simulink model "kukaXYZctrl"  (R2016b)
settings: Solver=ode5  StartTime=0.0  StopTime=inf  FixedStep=0.001  RelTol=1e-3  EnableMultiTasking=on
undefined symbols (not defined in the file): Standard_Devices, UDP_Protocol
libraries: dcpctrl x2, kukaslxctrl x1, sldrtlib x1, simulink x1
settings Model: SimulationMode=external  Creator=julianleland  LastModifiedBy=julianleland
settings OptimizationCC: LifeSpan=inf
settings DebuggingCC: SFUnexpectedBacktrackingDiag=warning  SFNoUnconditionalDefaultTransitionDiag=warning  SFExecutionAtInitializationDiag=none
settings HardwareCC: ProdBitPerLong=64  ProdHWDeviceType=Intel->x86-64 (Mac OS X)  TargetBitPerLong=64  TargetBitPerPointer=64  TargetIntDivRoundTo=Zero  TargetEndianess=LittleEndian  TargetWordSize=64  TargetHWDeviceType=Intel->x86-64
settings RTWCC: SystemTargetFile=sldrt.tlc  TemplateMakefile=sldrt.tmf  Description=Simulink Desktop Real-Time  RTWCompilerOptimization=on
settings CodeAppCC: MaxIdLength=95
settings SimulinkDesktopRealTimeCC: TargetPreCompLibLocation=/Applications/MATLAB_R2016b.app/toolbox/sldrt/lib/maci64  TargetLangStandard=C89/C90 (ANSI)  SupportVariableSizeSignals=off
settings ConfigComp: CovMetricSettings=dw  CovHtmlReporting=on  CovSaveCumulativeToWorkspaceVar=on  CovSaveSingleToWorkspaceVar=on  CovExternalEMLEnable=off

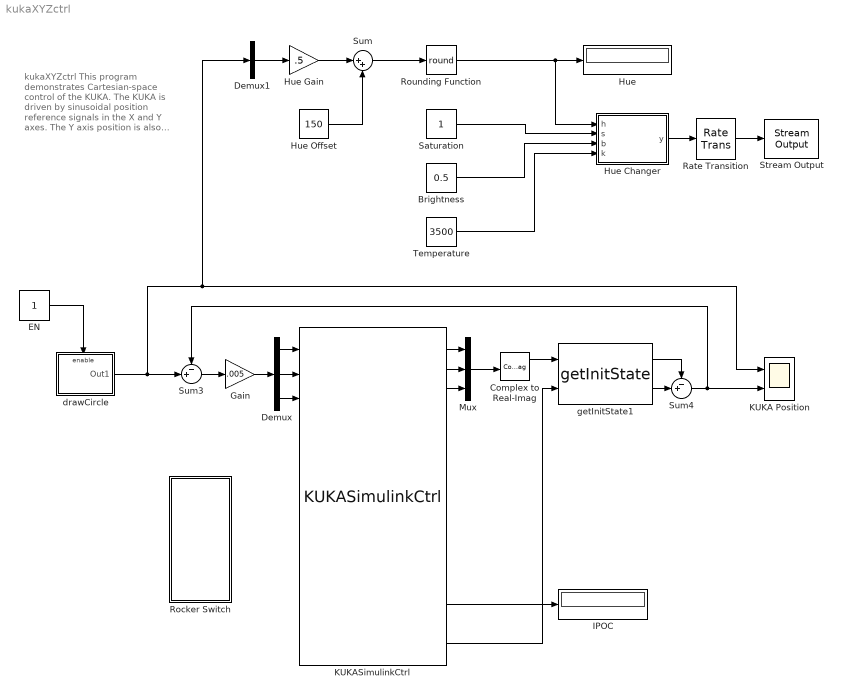
== system kukaXYZctrl ==
  note: kukaXYZctrl
      |
      | This program demonstrates Cartesian-space control of the KUKA. The KUKA is driven by sinusoidal position reference signals in the X and Y axes.
      |
      | The Y axis position is also used to drive the hue of the LIFX light-painting end-effector.
  Brightness : Constant  Value=0.5  OutMax=[1]  OutDataTypeStr=double
  Complex to Real-Imag : ComplexToRealImag
  Demux : Demux  Outputs=3
  Demux1 : Demux  Outputs=3
  EN : Constant
  Gain : Gain  Gain=.005
  Hue : Display
  Hue Changer : MATLAB Function  TreatAsAtomicUnit=on
  Hue Gain : Gain  Gain=.5
  Hue Offset : Constant  Value=150
  IPOC : Display
  KUKA Position : Scope  NumInputPorts=2
  KUKASimulinkCtrl : kukaslxctrl/KUKASimulinkCtrl
  Mux : Mux  Inputs=3
  Rate Transition : RateTransition
  Rocker Switch : Subsystem  DialogController=hmiCreateDDGDialog  IsWebBlock=on  mask(MWDashboardBlock){webBlockId=3e8c6259-59c1-4042-afd8-690274d47d06, webBlockType=rockerswitch, ShowInLibBrowser=on, ShowInitialText=on, HMISrcModelName=kukaXYZctrl}
      mask prompts: webBlockId "WebBlock Id"; webBlockType "WebBlock Type"; HMISrcModelName "Source Model"
      mask Help: helpview([docroot '/mapfiles/simulink.map'], 'hmi_rocker_switch')
      mask Display:
      | if strcmp(get_param(bdroot(gcb),'BlockDiagramType'), 'library')
      |     image([(matlabroot) '/toolbox/simulink/hmi/icons/RockerSwitch.png']);
      | end
  Rounding Function : Rounding  Operator=round
  Saturation : Constant  OutDataTypeStr=double
  Stream Output : sldrtlib/Stream Output  SampleTime=.1  MaxMissedTicks=10  ShowMissedTicks=off  YieldWhenWaiting=on  DrvName=Standard_Devices/UDP_Protocol  DrvAddress=54359  DrvOptions=[174338150 56700]  PortSizes=49  FormatString=repmat('%c',1,49)  ShowReady=off  ShowError=off  InitialValue=[]  FinalValue=[]
      settings: AttributesFormatString=Standard Devices\nUDP Protocol [D457h]
  Sum : Sum  Inputs=|++
  Sum3 : Sum  Inputs=-+|
  Sum4 : Sum  Inputs=-+|
  Temperature : Constant  Value=3500  OutMin=[2500]  OutMax=[9000]  OutDataTypeStr=double
  drawCircle : Subsystem
  getInitState1 : dcpctrl/getInitState
  wires:
  Sum3/1 -> Gain/1
  Gain/1 -> Demux/1
  Sum4/1 -> KUKA Position/2, Sum3/1
  Complex to Real-Imag/1 -> getInitState1/1
  getInitState1/2 -> Sum4/2
  getInitState1/1 -> Sum4/1
  KUKASimulinkCtrl/16 -> getInitState1/2
  KUKASimulinkCtrl/1 -> Mux/1
  KUKASimulinkCtrl/2 -> Mux/2
  KUKASimulinkCtrl/3 -> Mux/3
  Mux/1 -> Complex to Real-Imag/1
  Demux/1 -> KUKASimulinkCtrl/1
  Demux/2 -> KUKASimulinkCtrl/2
  Demux/3 -> KUKASimulinkCtrl/3
  drawCircle/1(Out1) -> KUKA Position/1, Demux1/1, Sum3/2
  EN/1 -> drawCircle/Enable
  KUKASimulinkCtrl/14 -> IPOC/1
  Hue Changer/1(y) -> Rate Transition/1
  Saturation/1 -> Hue Changer/2(s)
  Brightness/1 -> Hue Changer/3(b)
  Temperature/1 -> Hue Changer/4(k)
  Rounding Function/1 -> Hue/1, Hue Changer/1(h)
  Hue Gain/1 -> Sum/1
  Sum/1 -> Rounding Function/1
  Hue Offset/1 -> Sum/2
  Rate Transition/1 -> Stream Output/1
  Demux1/2 -> Hue Gain/1

== system kukaXYZctrl/Rocker Switch ==

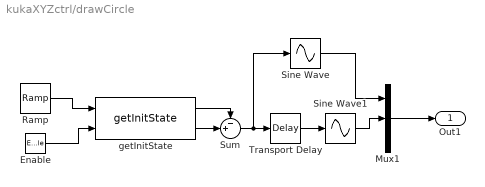
== system kukaXYZctrl/drawCircle ==
  Enable : EnablePort  ShowOutputPort=on
  Mux1 : Mux  Inputs=3
  Ramp : simulink/Sources/Ramp  slope=1  start=0  X0=0
  Sine Wave : Sin  TimeSource=Use external signal  Amplitude=200  Frequency=0.5  SampleTime=0
  Sine Wave1 : Sin  TimeSource=Use external signal  Amplitude=200  Frequency=0.5  SampleTime=0
  Sum : Sum  Inputs=-+|
  Transport Delay : TransportDelay  DelayTime=3
  getInitState : dcpctrl/getInitState
  Out1 : Outport
  wires:
  Sine Wave/1 -> Mux1/1
  Sine Wave1/1 -> Mux1/2
  Mux1/1 -> Out1/1
  Enable/1 -> getInitState/2
  Ramp/1 -> getInitState/1
  getInitState/2 -> Sum/2
  getInitState/1 -> Sum/1
  Sum/1 -> Transport Delay/1, Sine Wave/1
  Transport Delay/1 -> Sine Wave1/1

== matlab function kukaXYZctrl/Hue Changer ==
  data: h input; y output size=[1,49]; s input; b input; k input
function y = fcn(h,s,b,k)
%#codegen
%%
dec_code = [49;0;0;52;0;0;0;0;0;0;0;0;0;0;0;0;0;0;0;0;0;0;0;0;0;0;0;0;0;0;0;0;102;0;0;0;0;85;85;255;255;255;255;191;218;0;4;0;0];
%%
%%HUE 
hue = h/360 * 65535; %hue conversion formula, from degrees scale to LIFX scale
hue = floor(hue);
hue_hex = dec2hex(hue);

if (length(hue_hex) == 1)
    hue_arr = ['0',hue_hex(1)];
    hue_arr = ['00',hue_arr(1:2)];

elseif (length(hue_hex) ==2)
    hue_arr = ['00',hue_hex(1:2)];  
    
elseif (length(hue_hex) == 3)
    hue_arr = ['0', hue_hex(1), hue_hex(2), hue_hex(3)];
    hue_arr = [hue_arr(1:2),hue_arr(3:4)];
    
else
    hue_arr = [hue_hex(1:2), hue_hex(3:4)];
        
end

hue_out = hex2dec(hue_arr(1:2));
hue_out2 = hex2dec(hue_arr(3:4));

dec_code(38) = hue_out2;
dec_code(39) = hue_out;

%%
%SATURATION
sat = s * 65535; %saturation conversion formula, from 0-1 to LIFX scale
sat = floor(sat);
sat_hex = dec2hex(sat);

if (length(sat_hex) == 1)
    sat_arr = ['0',sat_hex(1)];
    sat_arr = ['00',sat_arr(1:2)];

elseif (length(sat_hex) ==2)
    sat_arr = ['00',sat_hex(1:2)];  
    
elseif (length(sat_hex) == 3)
    sat_arr = ['0', sat_hex(1), sat_hex(2), sat_hex(3)];
    sat_arr = [sat_arr(1:2),sat_arr(3:4)];
    
else
    sat_arr = [sat_hex(1:2), sat_hex(3:4)];
        
end

sat_out = hex2dec(sat_arr(1:2));
sat_out2 = hex2dec(sat_arr(3:4));

dec_code(40) = sat_out2;
dec_code(41) = sat_out;

%%

%BRIGHTNESS
bright = b * 65535; %brightness conversion formula, from 0-1 to LIFX scale
bright = floor(bright);
bright_hex = dec2hex(bright);

if (length(bright_hex) == 1)
    bright_arr = ['0',bright_hex(1)];
    bright_arr = ['00',bright_arr(1:2)];

elseif (length(bright_hex) ==2)
    bright_arr = ['00',bright_hex(1:2)];  
    
elseif (length(bright_hex) == 3)
    bright_arr = ['0', bright_hex(1), bright_hex(2), bright_hex(3)];
    bright_arr = [bright_arr(1:2),bright_arr(3:4)];
    
else
    bright_arr = [bright_hex(1:2), bright_hex(3:4)];
end

bright_out = hex2dec(bright_arr(1:2));
bright_out2 = hex2dec(bright_arr(3:4));

dec_code(42) = bright_out2;
dec_code(43) = bright_out;

%%
%KELVIN
kelvin = k; %Kelvin conversion formula, from 0-1 to LIFX scale
kelvin = floor(kelvin);
kelvin_hex = dec2hex(kelvin);

if (length(kelvin_hex) == 1)
    kelvin_arr = ['0',kelvin_hex(1)];
    kelvin_arr = ['00',kelvin_arr(1:2)];

elseif (length(kelvin_hex) ==2)
    kelvin_arr = ['00',kelvin_hex(1:2)];  
    
elseif (length(kelvin_hex) == 3)
    kelvin_arr = ['0', kelvin_hex(1), kelvin_hex(2), kelvin_hex(3)];
    kelvin_arr = [kelvin_arr(1:2), kelvin_arr(3:4)];
    
else
    kelvin_arr = [kelvin_hex(1:2), kelvin_hex(3:4)];
end

kelvin_out = hex2dec(kelvin_arr(1:2));
kelvin_out2 = hex2dec(kelvin_arr(3:4));

dec_code(44) = kelvin_out2;
dec_code(45) = kelvin_out;

%%
%y_temp = char_out;
%y = y_temp(1:2);

y = uint8(dec_code');
